simulink model "marieta"  (R2020a)
settings: Solver=VariableStepAuto  StartTime=0  StopTime=10  RelTol=1e-3
settings Model: Creator=Aro  LastModifiedBy=xacha

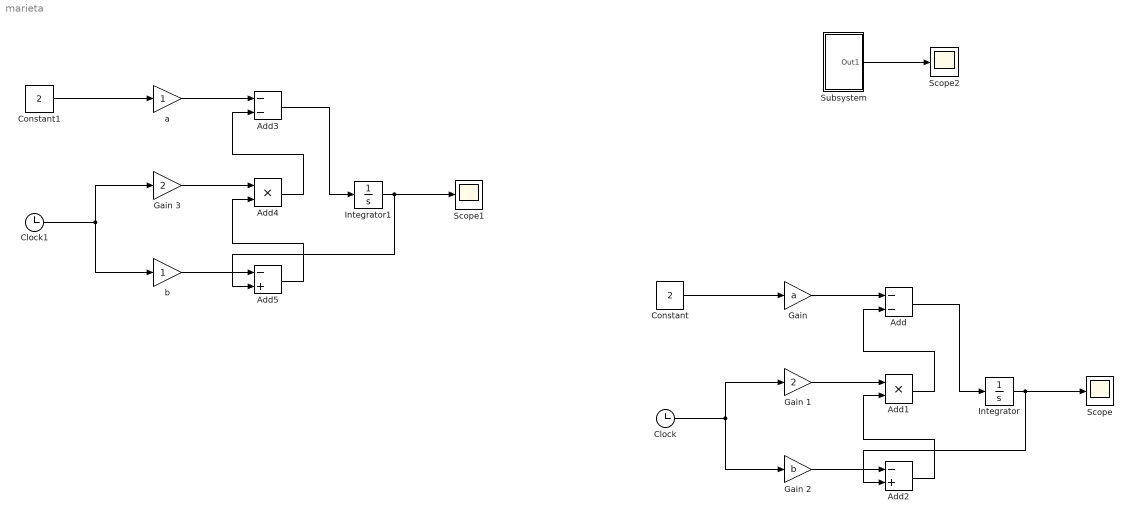
== system marieta ==
  Add : Sum  Inputs=--
  Add1 : Product
  Add2 : Sum  Inputs=-+
  Add3 : Sum  Inputs=--
  Add4 : Product
  Add5 : Sum  Inputs=-+
  Clock : Clock
  Clock1 : Clock
  Constant : Constant  Value=2
  Constant1 : Constant  Value=2
  Gain : Gain  Gain=a  mask{a=1}
      mask prompts: a "input a"
  Gain 1 : Gain  Gain=2
  Gain 2 : Gain  Gain=b  mask{b=1}
      mask prompts: b "input b"
  Gain 3 : Gain  Gain=2
  Integrator : Integrator  InitialCondition=2
  Integrator1 : Integrator  InitialCondition=2
  Scope : Scope
  Scope1 : Scope
  Scope2 : Scope
  Subsystem : Subsystem  mask{a=1, b=1}
      mask prompts: a "input a"; b "input b"
  a : Gain
  b : Gain
  wires:
  Clock/1 -> Gain 1/1, Gain 2/1
  Gain 2/1 -> Add2/1
  Integrator/1 -> Add2/2, Scope/1
  Add2/1 -> Add1/2
  Add1/1 -> Add/2
  Add/1 -> Integrator/1
  Gain 1/1 -> Add1/1
  Gain/1 -> Add/1
  Constant/1 -> Gain/1
  Constant1/1 -> a/1
  Add5/1 -> Add4/2
  Gain 3/1 -> Add4/1
  Clock1/1 -> b/1, Gain 3/1
  Add3/1 -> Integrator1/1
  a/1 -> Add3/1
  Add4/1 -> Add3/2
  b/1 -> Add5/1
  Integrator1/1 -> Add5/2, Scope1/1
  Subsystem/1(Out1) -> Scope2/1

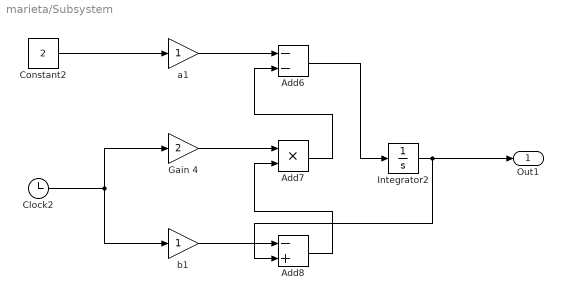
== system marieta/Subsystem ==
  Add6 : Sum  Inputs=--
  Add7 : Product
  Add8 : Sum  Inputs=-+
  Clock2 : Clock
  Constant2 : Constant  Value=2
  Gain 4 : Gain  Gain=2
  Integrator2 : Integrator  InitialCondition=2
  a1 : Gain
  b1 : Gain
  Out1 : Outport
  wires:
  Add8/1 -> Add7/2
  Add7/1 -> Add6/2
  Integrator2/1 -> Out1/1, Add8/2
  Clock2/1 -> b1/1, Gain 4/1
  b1/1 -> Add8/1
  Gain 4/1 -> Add7/1
  Constant2/1 -> a1/1
  Add6/1 -> Integrator2/1
  a1/1 -> Add6/1
